simulink subsystem "Tractor_mechanical"  (R2022b)
settings: Solver=VariableStepAuto  StartTime=0.0  StopTime=10.0  RelTol=1e-3
libraries: fl_lib x13, nesl_utility x9, sdl_lib x7, sh_lib x4, slpidlib x1
settings Model: Creator=david  LastModifiedBy=david

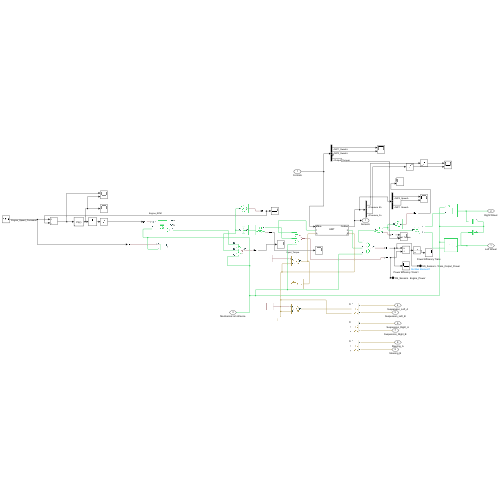
[thumbnail: Simulink's stored preview of the top-level diagram]
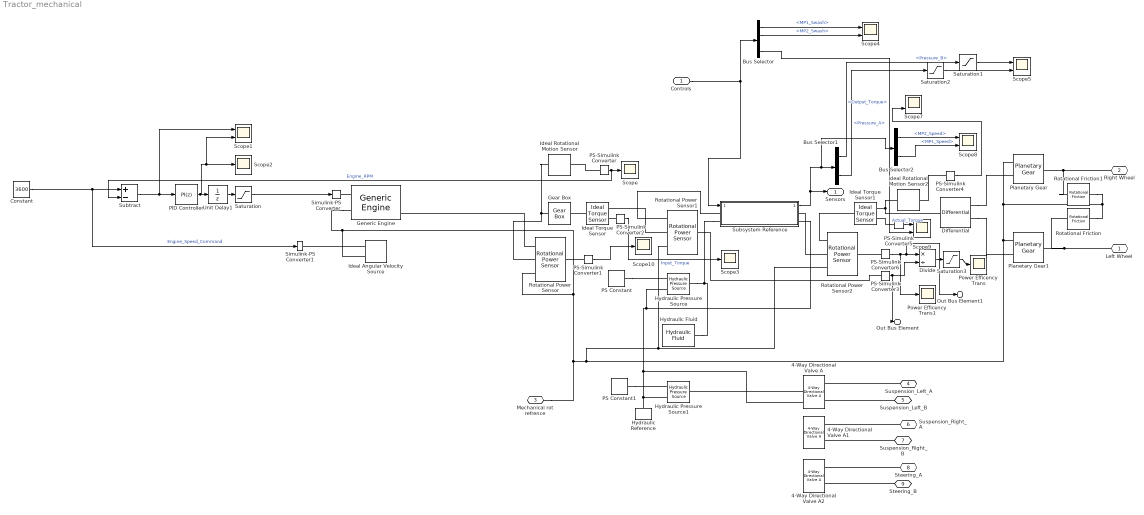
== system Tractor_mechanical ==
  Controls : Inport
  4-Way Directional Valve A : sh_lib/Valves/Directional Valves/4-Way Directional Valve A  mdl_type=1  area_max=.1 in^2  opening_max=10000 m  opening_tab=[-.002, 0, .002, .005, .015] m  area_tab=[1e-09, 2.0352e-07, 4.0736e-05, .00011438, .00034356] m^2  pressure_tab=[-10000000, -5000000, -2000000, 2000000, 5000000, 10000000] Pa  flow_rate_tab=[-1e-07, -7.0711e-08, -4.4721e-08, 4.4721e-08, 7.0711e-08, 1e-07; -2.0352e-05, -1.4391e-05, -9.1017e-06, 9.1017e-06, 1.4391e-05, 2.0352e-05; -.0040736, -.0028805, -.0018218, .0018218, .0028805, .0040736; -.011438, -.0080879, -.0051152, .0051152, .0080879, .011438; -.034356, -.024293, -.015364, .015364, .024293, .034356] m^3/s  interp_method=1  extrap_method=1  C_d=0.7  A_leak=1e-12 m^2  lam_spec=1  B_lam=0.999  Re_cr=12  x_0_P_A=-2.5e-3 m  x_0_P_B=-2.5e-3 m  x_0_A_T=-2.5e-3 m  x_0_B_T=-2.5e-3 m  x_0_P_T1=2.5e-3 m  x_0_T1_T=2.5e-3 m
      settings: InternalSimscapePortConfiguration="{\"Bottom\":[],\"Left\":[{\"id\":\"A\",\"label\":\"A\",\"type\":\"foundation.hydraulic.hydraulic\"},{\"id\":\"B\",\"label\":\"B\",\"type\":\"foundation.hydraulic.hydraulic\"}],\"Right\":[{\"id\":\"S\",\"label\":\"S\",\"type\":\"input\"},{\"id\":\"P\",\"label\":\"P\",\"type\":\"foundation.hydraulic.hydraulic\"},{\"id\":\"T\",\"label\":\"T\",\"type\":\"foundation.hydraulic.hydraulic\"}],\"Top\":[]}"
  4-Way Directional Valve A1 : sh_lib/Valves/Directional Valves/4-Way Directional Valve A  mdl_type=1  area_max=.1 in^2  opening_max=10000 m  opening_tab=[-.002, 0, .002, .005, .015] m  area_tab=[1e-09, 2.0352e-07, 4.0736e-05, .00011438, .00034356] m^2  pressure_tab=[-10000000, -5000000, -2000000, 2000000, 5000000, 10000000] Pa  flow_rate_tab=[-1e-07, -7.0711e-08, -4.4721e-08, 4.4721e-08, 7.0711e-08, 1e-07; -2.0352e-05, -1.4391e-05, -9.1017e-06, 9.1017e-06, 1.4391e-05, 2.0352e-05; -.0040736, -.0028805, -.0018218, .0018218, .0028805, .0040736; -.011438, -.0080879, -.0051152, .0051152, .0080879, .011438; -.034356, -.024293, -.015364, .015364, .024293, .034356] m^3/s  interp_method=1  extrap_method=1  C_d=0.7  A_leak=1e-12 m^2  lam_spec=1  B_lam=0.999  Re_cr=12  x_0_P_A=-2.5e-3 m  x_0_P_B=-2.5e-3 m  x_0_A_T=-2.5e-3 m  x_0_B_T=-2.5e-3 m  x_0_P_T1=2.5e-3 m  x_0_T1_T=2.5e-3 m
      settings: InternalSimscapePortConfiguration="{\"Bottom\":[],\"Left\":[{\"id\":\"A\",\"label\":\"A\",\"type\":\"foundation.hydraulic.hydraulic\"},{\"id\":\"B\",\"label\":\"B\",\"type\":\"foundation.hydraulic.hydraulic\"}],\"Right\":[{\"id\":\"S\",\"label\":\"S\",\"type\":\"input\"},{\"id\":\"P\",\"label\":\"P\",\"type\":\"foundation.hydraulic.hydraulic\"},{\"id\":\"T\",\"label\":\"T\",\"type\":\"foundation.hydraulic.hydraulic\"}],\"Top\":[]}"
  4-Way Directional Valve A2 : sh_lib/Valves/Directional Valves/4-Way Directional Valve A  mdl_type=1  area_max=.1 in^2  opening_max=10000 m  opening_tab=[-.002, 0, .002, .005, .015] m  area_tab=[1e-09, 2.0352e-07, 4.0736e-05, .00011438, .00034356] m^2  pressure_tab=[-10000000, -5000000, -2000000, 2000000, 5000000, 10000000] Pa  flow_rate_tab=[-1e-07, -7.0711e-08, -4.4721e-08, 4.4721e-08, 7.0711e-08, 1e-07; -2.0352e-05, -1.4391e-05, -9.1017e-06, 9.1017e-06, 1.4391e-05, 2.0352e-05; -.0040736, -.0028805, -.0018218, .0018218, .0028805, .0040736; -.011438, -.0080879, -.0051152, .0051152, .0080879, .011438; -.034356, -.024293, -.015364, .015364, .024293, .034356] m^3/s  interp_method=1  extrap_method=1  C_d=0.7  A_leak=1e-12 m^2  lam_spec=1  B_lam=0.999  Re_cr=12  x_0_P_A=-2.5e-3 m  x_0_P_B=-2.5e-3 m  x_0_A_T=-2.5e-3 m  x_0_B_T=-2.5e-3 m  x_0_P_T1=2.5e-3 m  x_0_T1_T=2.5e-3 m
      settings: InternalSimscapePortConfiguration="{\"Bottom\":[],\"Left\":[{\"id\":\"A\",\"label\":\"A\",\"type\":\"foundation.hydraulic.hydraulic\"},{\"id\":\"B\",\"label\":\"B\",\"type\":\"foundation.hydraulic.hydraulic\"}],\"Right\":[{\"id\":\"S\",\"label\":\"S\",\"type\":\"input\"},{\"id\":\"P\",\"label\":\"P\",\"type\":\"foundation.hydraulic.hydraulic\"},{\"id\":\"T\",\"label\":\"T\",\"type\":\"foundation.hydraulic.hydraulic\"}],\"Top\":[]}"
  Bus Selector : BusSelector  OutputSignals=Trans.MP1_Swash,Trans.MP2_Swash,Trans.Engine_Speed_CMD,Trans.Output_Torque
  Bus Selector1 : BusSelector  OutputSignals=Pressure_B,Pressure_A
  Bus Selector2 : BusSelector  OutputSignals=MP2_Speed,MP1_Speed
  Constant : Constant  Value=3600
  Differential : sdl_lib/Gears/Differential  driveshaft_location=sdl.enum.differential_orientation.right  cd_ratio=4.6  friction_model=sdl.enum.gear_friction.constant  efficiency=[.85, .92]  temperature_TLU=[280, 300, 320] K  efficiency_ss_TLU=[.95, .9, .85]  efficiency_cd_TLU=[.95, .9, .85]  pwr_thr=[.001, .001] W  mu_visc=[0, 0] N*m*s/rad  model_inertia=simscape.enum.onoff.off  carrier_inertia=0.001 kg*m^2  planet_inertia=0.001 kg*m^2  thermal_mass=50 J/K  T_init=300 K
  Divide : Product  Inputs=*/
  Gear Box : fl_lib/Mechanical/Mechanisms/Gear Box  ratio=4/3  t_in_specify=off  t_in_priority=None  t_in=0 N*m  t_in_nominal_specify=off  t_in_nominal_unit=N*m  t_in_nominal_value=1  t_out_specify=off  t_out_priority=None  t_out=0 N*m  t_out_nominal_specify=off  t_out_nominal_unit=N*m  t_out_nominal_value=1
  Generic Engine : sdl_lib/Engines & Motors/Generic Engine  input_type=sdl.enum.GenericEngineInputType.NormalizedThrottle  model_parameterization=sdl.enum.engineParameterization.torque  engine_type=sdl.enum.engineType.SI  Trq_max=380 N*m  w_Trq_max=4300 rpm  P_max=31 HP_DIN  w_P_max=3300 rpm  w_max=5000 rpm  w_min=500 rpm  w_tab=[2168,2494,3012,3218,3466,3524,3602,3608,4000,5000] rpm  trq_tab=[54,55.25,48.5,47,38,30.75,19,18,0.1,.1] lbf*ft  pwr_tab=[10, 30, 70, 110, 165, 190, 220, 230] kW  interp_method=simscape.enum.interpolation.smooth  w_thr=100 rpm  model_inertia=sdl.enum.model_inertia.on  inertia=.1 kg*m^2  initial_velocity=3000 rpm  model_time_constant=sdl.enum.lagOffOn.off  time_constant=0.2 s  initial_normalized_throttle=0  fc_model=sdl.enum.fuel_consumption_model.FuelOff  fc_per_rev=25 mg/rev  fc_w_tab=[1000, 2000, 3000, 4000, 5000, 6000] rpm  fc_trq_tab=[0, 80, 160, 200, 240, 320, 360, 400] N*m  fc_tab=[.5, .9, 1.4, 1.6, 1.9, 2.7, 3.4, 4.4; 1, 1.7, 2.7, 3.1, 3.6, 5, 6, 7.4; 1.4, 2.7, 4, 4.8, 5.6, 7.5, 8.5, 10.5; 2, 3.6, 5.8, 6.7, 8, 10.4, 11.7, 13.3; 2.5, 4.8, 7.9, 9.4, 10.8, 14, 16.2, 18.6; 3.1, 6, 10.3, 11.9, 13.8, 18.4, 22, 26.5] g/s  bmep_tab=[0, 250, 500, 625, 750, 1000, 1150, 1250] kPa  bsfc_tab=[410, 380, 300, 280, 270, 290, 320, 380; 410, 370, 290, 270, 260, 270, 285, 320; 415, 380, 290, 275, 265, 270, 270, 300; 420, 390, 310, 290, 285, 280, 280, 285; 430, 410, 340, 320, 310, 300, 310, 320; 450, 430, 370, 340, 330, 330, 350, 380] g/(hr*kW)  fc_interp_method=simscape.enum.interpolation.linear  displaced_volume=400 cm^3  rev_per_cycle=2  idle_speed=true  idle_speed_reference=1000 rpm  tau_controller=1 s  idle_w_thr=1 rpm  redline=true  redline_speed=3600 rpm  tau_redline=1 s  redline_w_thr=1 rpm
      settings: InternalSimscapePortConfiguration="{\"Bottom\":[],\"Left\":[{\"id\":\"ThrNorm\",\"label\":\"Thr\",\"type\":\"input\"},{\"id\":\"B\",\"label\":\"B\",\"type\":\"foundation.mechanical.rotational.rotational\"}],\"Right\":[{\"id\":\"P\",\"label\":\"P\",\"type\":\"output\"},{\"id\":\"FC\",\"label\":\"FC\",\"type\":\"output\"},{\"id\":\"F\",\"label\":\"F\",\"type\":\"foundation.mechanical.rotational.rotational\"}],\"Top\":[]}"
  Hydraulic Fluid : sh_lib/Hydraulic Utilities/Hydraulic Fluid  SelFluid=15  SysTemp=60  TrapAir=0.005  ViscDerFactor=1  range_error=2
  Hydraulic Pressure Source : fl_lib/Hydraulic/Hydraulic Sources/Hydraulic Pressure Source
      settings: InternalSimscapePortConfiguration="{\"Bottom\":[],\"Left\":[{\"id\":\"P\",\"label\":\"P\",\"type\":\"foundation.hydraulic.hydraulic\"}],\"Right\":[{\"id\":\"S\",\"label\":\"S\",\"type\":\"input\"},{\"id\":\"T\",\"label\":\"T\",\"type\":\"foundation.hydraulic.hydraulic\"}],\"Top\":[]}"
  Hydraulic Pressure Source1 : fl_lib/Hydraulic/Hydraulic Sources/Hydraulic Pressure Source
      settings: InternalSimscapePortConfiguration="{\"Bottom\":[],\"Left\":[{\"id\":\"P\",\"label\":\"P\",\"type\":\"foundation.hydraulic.hydraulic\"}],\"Right\":[{\"id\":\"S\",\"label\":\"S\",\"type\":\"input\"},{\"id\":\"T\",\"label\":\"T\",\"type\":\"foundation.hydraulic.hydraulic\"}],\"Top\":[]}"
  Hydraulic Reference : fl_lib/Hydraulic/Hydraulic Elements/Hydraulic Reference
  Ideal Angular Velocity Source : fl_lib/Mechanical/Mechanical Sources/Ideal Angular Velocity Source
  Ideal Rotational Motion Sensor : fl_lib/Mechanical/Mechanical Sensors/Ideal Rotational Motion Sensor  reference=foundation.enum.MeasurementReference.absolute  acceleration_port=false  velocity_port=true  position_port=false  wrap_angle=false  offset=0 rad
      settings: InternalSimscapePortConfiguration="{\"Bottom\":[],\"Left\":[{\"id\":\"R\",\"label\":\"R\",\"type\":\"foundation.mechanical.rotational.rotational\"}],\"Right\":[{\"id\":\"W\",\"label\":\"W\",\"type\":\"output\"}],\"Top\":[]}"
  Ideal Rotational Motion Sensor2 : fl_lib/Mechanical/Mechanical Sensors/Ideal Rotational Motion Sensor  reference=foundation.enum.MeasurementReference.absolute  acceleration_port=false  velocity_port=true  position_port=false  wrap_angle=false  offset=0 rad
      settings: InternalSimscapePortConfiguration="{\"Bottom\":[],\"Left\":[{\"id\":\"R\",\"label\":\"R\",\"type\":\"foundation.mechanical.rotational.rotational\"}],\"Right\":[{\"id\":\"W\",\"label\":\"W\",\"type\":\"output\"}],\"Top\":[]}"
  Ideal Torque Sensor : fl_lib/Mechanical/Mechanical Sensors/Ideal Torque Sensor
  Ideal Torque Sensor1 : fl_lib/Mechanical/Mechanical Sensors/Ideal Torque Sensor
  PID Controller : slpidlib/PID Controller  Controller=PI  Form=Parallel  TimeDomain=Discrete-time  UseExternalTs=off  SampleTime=-1  IntegratorMethod=Forward Euler  FilterMethod=Forward Euler  ControllerParametersSource=internal  P=0.000362985474512188  I=2.4202875360901e-04  UseKiTs=off  D=0  N=100  UseFilter=on  TunerSelectOption=Transfer Function Based (PID Tuner App)  InitialConditionSource=internal  InitialConditionForIntegrator=0  InitialConditionForFilter=0  DifferentiatorICPrevScaledInput=0  ExternalReset=none  TrackingMode=off  Kt=1  LimitOutput=off  SatLimitsSource=internal  UpperSaturationLimit=inf  LowerSaturationLimit=-inf  LinearizeAsGain=on  AntiWindupMode=none  Kb=1  LimitIntegrator=off  UpperIntegratorSaturationLimit=inf  LowerIntegratorSaturationLimit=-inf  POutMin=[]  POutMax=[]  IOutMin=[]  IOutMax=[]  DOutMin=[]  DOutMax=[]  NOutMin=[]  NOutMax=[]  SumOutMin=[]  SumOutMax=[]  SaturationOutMin=[]  SaturationOutMax=[]  PParamMin=[]  PParamMax=[]  IParamMin=[]  IParamMax=[]  DParamMin=[]  DParamMax=[]  NParamMin=[]  NParamMax=[]  KbParamMin=[]  KbParamMax=[]  KtParamMin=[]  KtParamMax=[]  KbOutMin=[]  KbOutMax=[]  KtOutMin=[]  KtOutMax=[]  IntegratorOutMin=[]  IntegratorOutMax=[]  FilterOutMin=[]  FilterOutMax=[]  SumI1OutMin=[]  SumI1OutMax=[]  SumI2OutMin=[]  SumI2OutMax=[]  SumI3OutMin=[]  SumI3OutMax=[]  SumI4OutMin=[]  SumI4OutMax=[]  SumDOutMin=[]  SumDOutMax=[]  DifferentiatorOutMin=[]  DifferentiatorOutMax=[]  FilterDiffOutCoefMin=[]  FilterDiffOutCoefMax=[]  ReciprocalOutMin=[]  ReciprocalOutMax=[]  SumDenOutMin=[]  SumDenOutMax=[]  SumNumOutMin=[]  SumNumOutMax=[]  DivideOutMin=[]  DivideOutMax=[]  UdiffTsProdOutMin=[]  UdiffTsProdOutMax=[]  NTsProdOutMin=[]  NTsProdOutMax=[]  UintegralTsProdOutMin=[]  UintegralTsProdOutMax=[]  UngainTsProdOutMin=[]  UngainTsProdOutMax=[]  ClampingZeroOutDataTypeStr=Inherit: Inherit via back propagation  ClampingZeroOutMin=[]  ClampingZeroOutMax=[]  FilterDenConstantOutDataTypeStr=Inherit: Inherit via back propagation  FilterDenConstantOutMin=[]  FilterDenConstantOutMax=[]  PCopyOutDataTypeStr=Inherit: Inherit via back propagation  PCopyOutMin=[]  PCopyOutMax=[]  NCopyOutDataTypeStr=Inherit: Inherit via back propagation  NCopyOutMin=[]  NCopyOutMax=[]  IntegratorContinuousStateAttributes=''  IntegratorStateMustResolveToSignalObject=off  IntegratorRTWStateStorageClass=Auto  FilterContinuousStateAttributes=''  FilterStateMustResolveToSignalObject=off  FilterRTWStateStorageClass=Auto  ParallelPVariant=InternalParameters  IdealPVariant=Disabled  IVariant=InternalParameters  DVariant=Disabled  IntegratorVariant=Discrete  SatVariant=Disabled  AWVariant=Passthrough  PCopyVariant=Disabled  TRVariant=Disabled  FdbkBlocksVariant=Forward  IdealPFdbkVariant=Disabled  SatFdbkVariant=Disabled  DerivativeFilterVariant=Disabled  NVariant=Disabled  NCopyVariant=Disabled_SignalSpec  FilterICVariant=Disabled  IntegratorICVariant=InternalICs  ExternalResetVariant=Disabled  TRSumVariant=Passthrough  SumFdbkVariant=Disabled  SumVariant=Sum_PI  TsampFilterVariant=InternalTs  TsampNgainVariant=Passthrough  TsampIntegralVariant=Passthrough  ExternalSaturationOutDataTypeStr=Inherit: Same as second input
  PS Constant : fl_lib/Physical Signals/Sources/PS Constant  constant=150 psi
  PS Constant1 : fl_lib/Physical Signals/Sources/PS Constant  constant=1000 psi
  PS-Simulink Converter : nesl_utility/PS-Simulink Converter  PhysicalDomain=network_engine_domain  SubClassName=ps_output  LeftPortType=input  RightPortType=output  PseudoPeriodic=off  Frequencies=[]  VectorFormat=inherit  Unit=rpm  AffineConversion=off
  PS-Simulink Converter1 : nesl_utility/PS-Simulink Converter  PhysicalDomain=network_engine_domain  SubClassName=ps_output  LeftPortType=input  RightPortType=output  PseudoPeriodic=off  Frequencies=[]  VectorFormat=inherit  Unit=HP_DIN  AffineConversion=off
  PS-Simulink Converter2 : nesl_utility/PS-Simulink Converter  PhysicalDomain=network_engine_domain  SubClassName=ps_output  LeftPortType=input  RightPortType=output  PseudoPeriodic=off  Frequencies=[]  VectorFormat=inherit  Unit=ft*lb  AffineConversion=off
  PS-Simulink Converter3 : nesl_utility/PS-Simulink Converter  PhysicalDomain=network_engine_domain  SubClassName=ps_output  LeftPortType=input  RightPortType=output  PseudoPeriodic=off  Frequencies=[]  VectorFormat=inherit  Unit=inherit  AffineConversion=off
  PS-Simulink Converter4 : nesl_utility/PS-Simulink Converter  PhysicalDomain=network_engine_domain  SubClassName=ps_output  LeftPortType=input  RightPortType=output  PseudoPeriodic=off  Frequencies=[]  VectorFormat=inherit  Unit=rpm  AffineConversion=off
  PS-Simulink Converter5 : nesl_utility/PS-Simulink Converter  PhysicalDomain=network_engine_domain  SubClassName=ps_output  LeftPortType=input  RightPortType=output  PseudoPeriodic=off  Frequencies=[]  VectorFormat=inherit  Unit=ft*lb  AffineConversion=off
  PS-Simulink Converter6 : nesl_utility/PS-Simulink Converter  PhysicalDomain=network_engine_domain  SubClassName=ps_output  LeftPortType=input  RightPortType=output  PseudoPeriodic=off  Frequencies=[]  VectorFormat=inherit  Unit=inherit  AffineConversion=off
  Planetary Gear : sdl_lib/Gears/Planetary Gear  rs_ratio=2.81  friction_model=sdl.enum.gear_friction.constant  efficiency=[.96, .98]  temperature_TLU=[280, 300, 320] K  efficiency_sp_TLU=[.95, .9, .85]  efficiency_rp_TLU=[.95, .9, .85]  pwr_thr=[.001, .001] W  mu_visc=[0, 0] N*m*s/rad  model_inertia=simscape.enum.onoff.off  planet_inertia=0.001 kg*m^2  thermal_mass=50 J/K  T_init=300 K
  Planetary Gear1 : sdl_lib/Gears/Planetary Gear  rs_ratio=2.81  friction_model=sdl.enum.gear_friction.constant  efficiency=[.96, .98]  temperature_TLU=[280, 300, 320] K  efficiency_sp_TLU=[.95, .9, .85]  efficiency_rp_TLU=[.95, .9, .85]  pwr_thr=[.001, .001] W  mu_visc=[0, 0] N*m*s/rad  model_inertia=simscape.enum.onoff.off  planet_inertia=0.001 kg*m^2  thermal_mass=50 J/K  T_init=300 K
  Power Efficency Trans : Scope
  Power Efficency Trans1 : Scope
  Rotational Friction : fl_lib/Mechanical/Rotational Elements/Rotational Friction  brkwy_trq=10 lbf*ft  brkwy_vel=0.1 rad/s  Col_trq=5 lbf*ft  visc_coef=0.001 N*m*s/rad  w_specify=off  w_priority=None  w=0 rad/s  w_nominal_specify=off  w_nominal_unit=rad/s  w_nominal_value=1  t_specify=off  t_priority=None  t=0 N*m  t_nominal_specify=off  t_nominal_unit=N*m  t_nominal_value=1
  Rotational Friction1 : fl_lib/Mechanical/Rotational Elements/Rotational Friction  brkwy_trq=10 lbf*ft  brkwy_vel=0.1 rad/s  Col_trq=5 lbf*ft  visc_coef=0.001 N*m*s/rad  w_specify=off  w_priority=None  w=0 rad/s  w_nominal_specify=off  w_nominal_unit=rad/s  w_nominal_value=1  t_specify=off  t_priority=None  t=0 N*m  t_nominal_specify=off  t_nominal_unit=N*m  t_nominal_value=1
  Rotational Power Sensor : sdl_lib/Sensors/Rotational Power Sensor  measurement_type=sdl.enum.rotationalPowerSensorType.instantaneous  averaging_period=1 s  max_frequency=1000 Hz  max_speed=1000 rpm
      settings: InternalSimscapePortConfiguration="{\"Bottom\":[],\"Left\":[{\"id\":\"S\",\"label\":\"S\",\"type\":\"foundation.mechanical.rotational.rotational\"},{\"id\":\"R\",\"label\":\"R\",\"type\":\"foundation.mechanical.rotational.rotational\"},{\"id\":\"C\",\"label\":\"C\",\"type\":\"foundation.mechanical.rotational.rotational\"}],\"Right\":[{\"id\":\"P\",\"label\":\"P\",\"type\":\"output\"}],\"Top\":[]}"
  Rotational Power Sensor1 : sdl_lib/Sensors/Rotational Power Sensor  measurement_type=sdl.enum.rotationalPowerSensorType.instantaneous  averaging_period=1 s  max_frequency=1000 Hz  max_speed=1000 rpm
      settings: InternalSimscapePortConfiguration="{\"Bottom\":[],\"Left\":[{\"id\":\"S\",\"label\":\"S\",\"type\":\"foundation.mechanical.rotational.rotational\"},{\"id\":\"R\",\"label\":\"R\",\"type\":\"foundation.mechanical.rotational.rotational\"},{\"id\":\"C\",\"label\":\"C\",\"type\":\"foundation.mechanical.rotational.rotational\"}],\"Right\":[{\"id\":\"P\",\"label\":\"P\",\"type\":\"output\"}],\"Top\":[]}"
  Rotational Power Sensor2 : sdl_lib/Sensors/Rotational Power Sensor  measurement_type=sdl.enum.rotationalPowerSensorType.instantaneous  averaging_period=1 s  max_frequency=1000 Hz  max_speed=1000 rpm
      settings: InternalSimscapePortConfiguration="{\"Bottom\":[],\"Left\":[{\"id\":\"S\",\"label\":\"S\",\"type\":\"foundation.mechanical.rotational.rotational\"},{\"id\":\"R\",\"label\":\"R\",\"type\":\"foundation.mechanical.rotational.rotational\"},{\"id\":\"C\",\"label\":\"C\",\"type\":\"foundation.mechanical.rotational.rotational\"}],\"Right\":[{\"id\":\"P\",\"label\":\"P\",\"type\":\"output\"}],\"Top\":[]}"
  Saturation : Saturate  UpperLimit=01  LowerLimit=0
  Saturation1 : Saturate  UpperLimit=20000  LowerLimit=0
  Saturation2 : Saturate  UpperLimit=20000  LowerLimit=0
  Saturation3 : Saturate  UpperLimit=1  LowerLimit=0
  Scope{,2..3,10} (4 alike) : Scope
  Scope{1,4..5,7..9} (6 alike) : Scope  NumInputPorts=2
  Simulink-PS Converter : nesl_utility/Simulink-PS Converter  PhysicalDomain=network_engine_domain  SubClassName=ps_input  LeftPortType=input  RightPortType=output  PseudoPeriodic=off  Frequencies=[]  NoiseDistribution=none  NoiseParameters=[]  Unit=1  AffineConversion=off  FilteringAndDerivatives=provide  SimscapeFilterOrder=1  InputFilterTimeConstant=0.001  UdotUserProvided=0
  Simulink-PS Converter1 : nesl_utility/Simulink-PS Converter  PhysicalDomain=network_engine_domain  SubClassName=ps_input  LeftPortType=input  RightPortType=output  PseudoPeriodic=off  Frequencies=[]  NoiseDistribution=none  NoiseParameters=[]  Unit=rpm  AffineConversion=off  FilteringAndDerivatives=provide  SimscapeFilterOrder=1  InputFilterTimeConstant=0.001  UdotUserProvided=0
  Subsystem Reference : Subsystem  ReferencedSubsystem=HMT
      settings: PortSchema="{\"entries\":[{\"content\":{\"sides\":[{\"content\":{\"connectorIds\":[\"In1\",\"RConn1\",\"LConn2\"]},\"type\":\"ConnectorPlacement.EquallySpacedRectSide\",\"uuid\":\"fdedb491-33de-44d0-87bf-4d938b73adb2\"},{\"content\":{\"connectorIds\":[\"Out1\",\"LConn1\",\"RConn2\"],\"side\":\"RIGHT\"},\"type\":\"ConnectorPlacement.EquallySpacedRectSide\",\"uuid\":\"846da588-6b34-4f0a-8826-c79aa7268cc7\"},{\"content\":{\"connectorIds\":[],\"side\":\"TOP\"},\"type\":\"ConnectorPlacement.EquallySpacedRectSide\",\"uuid\":\"12499447-05b1-4785-87b7-03b761060a74\"}]},\"type\":\"ConnectorPlacement.EquallySpacedConnector\",\"uuid\":\"53284d45-9163-442b-91da-45ee3b70adf9\"}],\"packageUris\":[\"http://schema.mathworks.com/mf0/Connector/R2020b\"],\"version\":\"1.0\"}"
  Subtract : Sum  Inputs=+-
  Unit Delay1 : UnitDelay  SampleTime=-1  HasFrameUpgradeWarning=on
  Left Wheel : PMIOPort  Side=Right
  Right Wheel : PMIOPort  Port=2  Side=Right
  Mechanical rot refrence : PMIOPort  Port=3  Side=Left
  Suspension_Left_A : PMIOPort  Port=4  Side=Right
  Suspension_Left_B : PMIOPort  Port=5  Side=Right
  Suspension_Right_A : PMIOPort  Port=6  Side=Right
  Suspension_Right_B : PMIOPort  Port=7  Side=Right
  Steering_A : PMIOPort  Port=8  Side=Right
  Steering_B : PMIOPort  Port=9  Side=Right
  Sensors : Outport
  Out Bus Element : Outport  Port=2  PortName=SS_Sensors  Element=Engine_Power
  Out Bus Element1 : Outport  Port=2  PortName=SS_Sensors  Element=Trans_Output_Power
  wires:
  PS-Simulink Converter4/1 -> Scope7/2
  Subsystem Reference/1 -> Sensors/1, Bus Selector1/1, Bus Selector2/1
  Bus Selector/1 -> Scope4/1  "<MP1_Swash>"
  Bus Selector2/2 -> Scope8/2  "<MP1_Speed>"
  PS-Simulink Converter/1 -> Scope/1, Subtract/2  "Engine_RPM"
  Constant/1 -> Subtract/1, Simulink-PS Converter1/1  "Engine_Speed_Command"
  Subtract/1 -> Scope1/1, PID Controller/1
  PS-Simulink Converter6/1 -> Out Bus Element1/1, Divide/1, Power Efficency Trans1/1
  Bus Selector/2 -> Scope4/2  "<MP2_Swash>"
  Bus Selector1/2 -> Saturation2/1  "<Pressure_A>"
  Saturation2/1 -> Scope5/2
  PS-Simulink Converter2/1 -> Scope3/1  "Input_Torque"
  Saturation/1 -> Simulink-PS Converter/1
  PID Controller/1 -> Unit Delay1/1, Scope1/2, Scope2/1
  Controls/1 -> Bus Selector/1, Subsystem Reference/1
  PS-Simulink Converter5/1 -> Scope9/1  "Actual_Torque"
  Bus Selector1/1 -> Saturation1/1  "<Pressure_B>"
  PS-Simulink Converter1/1 -> Scope10/1
  Bus Selector/4 -> Scope9/2  "<Output_Torque>"
  Bus Selector2/1 -> Scope8/1  "<MP2_Speed>"
  Divide/1 -> Saturation3/1
  Saturation3/1 -> Power Efficency Trans/1
  Saturation1/1 -> Scope5/1
  PS-Simulink Converter3/1 -> Out Bus Element/1, Divide/2
  Unit Delay1/1 -> Saturation/1
  connections:
  Generic Engine/LConn2 -- Rotational Friction/RConn1 -- Rotational Friction1/RConn1 -- Planetary Gear/RConn1 -- Planetary Gear1/RConn1 -- Rotational Power Sensor1/LConn3 -- Rotational Power Sensor2/LConn3 -- Mechanical rot refrence/RConn1 -- Rotational Power Sensor/LConn3 -- Ideal Angular Velocity Source/RConn2
  Subsystem Reference/LConn2 -- Hydraulic Fluid/RConn1 -- Hydraulic Pressure Source/LConn1
  Gear Box/LConn1 -- Rotational Power Sensor/LConn2 -- Ideal Rotational Motion Sensor/LConn1
  Ideal Torque Sensor1/RConn1 -- Differential/LConn1 -- Ideal Rotational Motion Sensor2/LConn1
  Hydraulic Pressure Source1/RConn2 -- Subsystem Reference/RConn2 -- Hydraulic Pressure Source/RConn2 -- 4-Way Directional Valve A/RConn3 -- Hydraulic Reference/LConn1
  Planetary Gear1/LConn1 -- Rotational Friction/LConn1 -- Left Wheel/RConn1
  Planetary Gear/LConn1 -- Rotational Friction1/LConn1 -- Right Wheel/RConn1
  Rotational Power Sensor2/LConn2 -- Subsystem Reference/LConn1
  Rotational Power Sensor/LConn1 -- Generic Engine/RConn3
  PS-Simulink Converter6/LConn1 -- Rotational Power Sensor2/RConn1
  PS-Simulink Converter2/LConn1 -- Ideal Torque Sensor/RConn2
  PS Constant/RConn1 -- Hydraulic Pressure Source/RConn1
  Ideal Torque Sensor/LConn1 -- Gear Box/RConn1
  Generic Engine/LConn1 -- Simulink-PS Converter/RConn1
  Ideal Angular Velocity Source/RConn1 -- Simulink-PS Converter1/RConn1
  PS-Simulink Converter1/LConn1 -- Rotational Power Sensor/RConn1
  Differential/RConn1 -- Planetary Gear/RConn2
  PS-Simulink Converter3/LConn1 -- Rotational Power Sensor1/RConn1
  Rotational Power Sensor1/LConn1 -- Subsystem Reference/RConn1
  Rotational Power Sensor1/LConn2 -- Ideal Torque Sensor/RConn1
  PS-Simulink Converter5/LConn1 -- Ideal Torque Sensor1/RConn2
  PS-Simulink Converter/LConn1 -- Ideal Rotational Motion Sensor/RConn1
  PS-Simulink Converter4/LConn1 -- Ideal Rotational Motion Sensor2/RConn1
  Differential/RConn2 -- Planetary Gear1/RConn2
  Rotational Power Sensor2/LConn1 -- Ideal Torque Sensor1/LConn1
  PS Constant1/RConn1 -- Hydraulic Pressure Source1/RConn1
  4-Way Directional Valve A/RConn2 -- Hydraulic Pressure Source1/LConn1
  Suspension_Left_B/RConn1 -- 4-Way Directional Valve A/LConn2
  Suspension_Left_A/RConn1 -- 4-Way Directional Valve A/LConn1
  Suspension_Right_A/RConn1 -- 4-Way Directional Valve A1/LConn1
  Suspension_Right_B/RConn1 -- 4-Way Directional Valve A1/LConn2
  Steering_A/RConn1 -- 4-Way Directional Valve A2/LConn1
  Steering_B/RConn1 -- 4-Way Directional Valve A2/LConn2
